simulink model "Airbag_donePrev"  (R2020b)
settings: Solver=VariableStepAuto  StartTime=0.0  StopTime=10  RelTol=1e-3
libraries: simulink x4
settings Model: Creator=HP  LastModifiedBy=HP

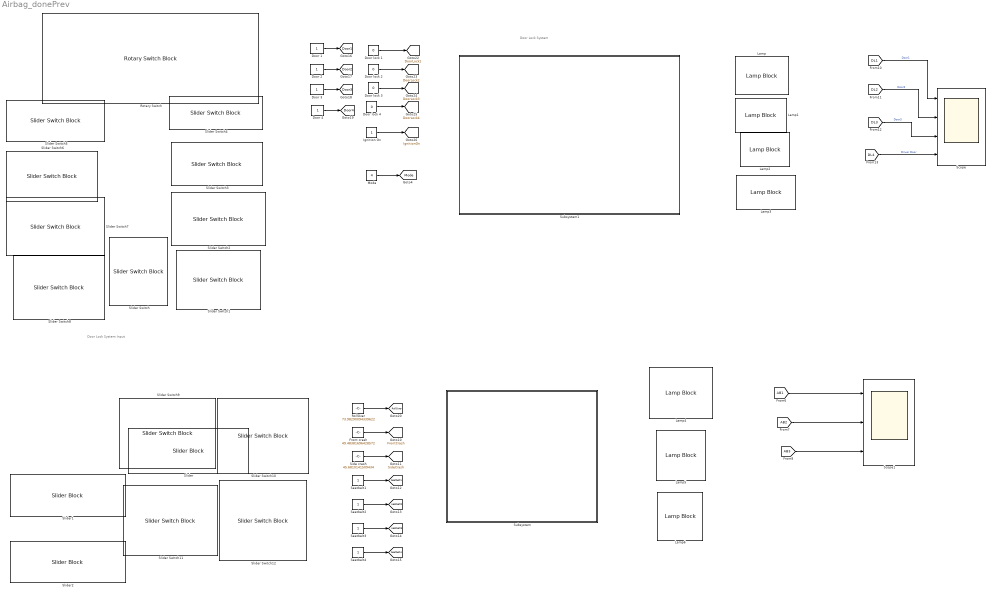
== system Airbag_donePrev ==
  note: Door Lock System
  note: Door Lock System Input
  Door {1..4} (4 alike) : Constant
  Door lock {1..4} (4 alike) : Constant  Value=0
  Front crash : Constant  Value=49.48381696428572
  Ignition On : Constant
  Lamp{,1..6} (7 alike) : LampBlock
  Mode : Constant  Value=4
  RollOver : Constant  Value=73.98290094339622
  Rotary Switch : RotarySwitchBlock
      settings: Values={{'Safety lock', 'Automatic Lock', 'Lock Out Protection', 'Driver Control Lock', 'Driver Control Unlock'}, [0 1 2 3 4]}
  Scope : Scope  NumInputPorts=4
  Scope1 : Scope  NumInputPorts=3
  Seatbelt{1..4} (4 alike) : Constant
  Side crash : Constant  Value=45.6810141509434
  Slider : SliderBlock
  Slider Switch{,1..12} (13 alike) : SliderSwitchBlock
      settings: Values={{'Off', 'On'}, [0 1]}
  Slider1 : SliderBlock
  Slider2 : SliderBlock
  Subsystem : Subsystem
  Subsystem1 : Subsystem
  tag scope: Door1=global, Door2=global, Door3=global, Door4=global, DoorLock1=global, DoorLock2=global, DoorLock3=global, DoorLock4=global, FrontCrash=global, IgnitionOn=global, Mode=global, RollOver=global, Seatbelt1=global, Seatbelt4=global, SideCrash=global, seatbelt2=global, seatbelt3=global
  wires:
  RollOver/1 -> [RollOver]
  Seatbelt3/1 -> [seatbelt3]
  Mode/1 -> [Mode]
  Seatbelt4/1 -> [Seatbelt4]
  Seatbelt2/1 -> [seatbelt2]
  [DL1] -> Scope/1  "Door1"
  Seatbelt1/1 -> [Seatbelt1]
  [DL4] -> Scope/4  "Driver Door"
  Side crash/1 -> [SideCrash]
  [DL2] -> Scope/2  "Door2"
  [AB1] -> Scope1/1
  [DL3] -> Scope/3  "Door3"
  [AB3] -> Scope1/3
  Front crash/1 -> [FrontCrash]
  [AB2] -> Scope1/2
  Door 3/1 -> [Door3]
  Ignition On/1 -> [IgnitionOn]
  Door lock 2/1 -> [DoorLock2]
  Door lock 3/1 -> [DoorLock3]
  Door lock 1/1 -> [DoorLock1]
  Door lock 4/1 -> [DoorLock4]
  Door 1/1 -> [Door1]
  Door 2/1 -> [Door2]
  Door 4/1 -> [Door4]

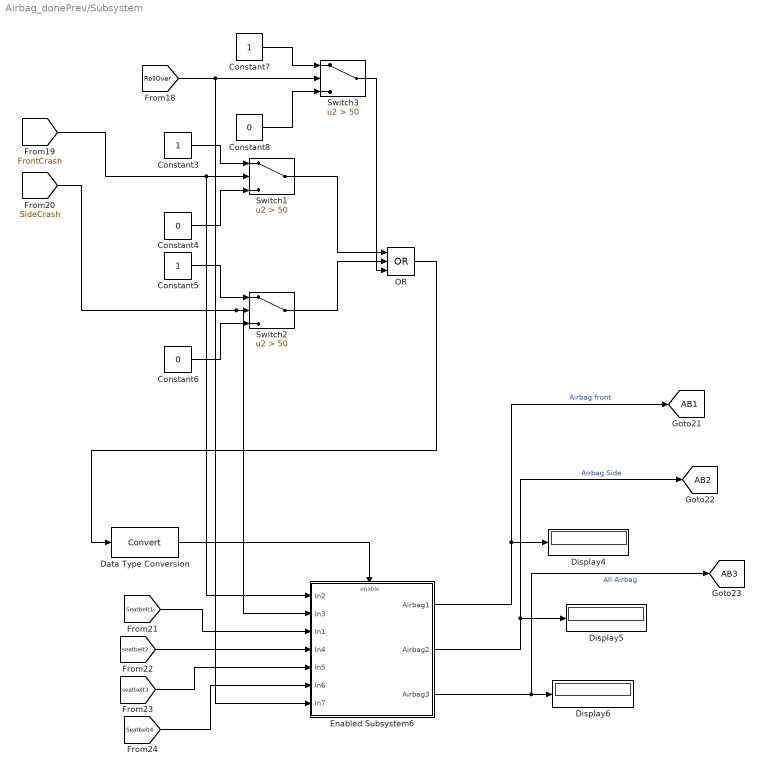
== system Airbag_donePrev/Subsystem ==
  Constant3 : Constant
  Constant4 : Constant  Value=0
  Constant5 : Constant
  Constant6 : Constant  Value=0
  Constant7 : Constant
  Constant8 : Constant  Value=0
  Data Type Conversion : DataTypeConversion
  Display4 : Display
  Display5 : Display
  Display6 : Display
  Enabled Subsystem6 : Subsystem  TreatAsAtomicUnit=on
  OR : Logic  Operator=OR  Inputs=3  IconShape=distinctive  AllPortsSameDT=off  OutDataTypeStr=boolean
  Switch1 : Switch  Criteria=u2 > Threshold  Threshold=50
  Switch2 : Switch  Criteria=u2 > Threshold  Threshold=50
  Switch3 : Switch  Criteria=u2 > Threshold  Threshold=50
  tag scope: AB1=global, AB2=global, AB3=global
  wires:
  Enabled Subsystem6/2(Airbag2) -> [AB2], Display5/1  "Airbag Side"
  Constant7/1 -> Switch3/1
  [Seatbelt4] -> Enabled Subsystem6/6(In6)
  Enabled Subsystem6/3(Airbag3) -> [AB3], Display6/1  "All Airbag"
  [RollOver] -> Enabled Subsystem6/7(In7), Switch3/2
  [seatbelt3] -> Enabled Subsystem6/5(In5)
  [SideCrash] -> Enabled Subsystem6/2(In3), Switch2/2
  Enabled Subsystem6/1(Airbag1) -> [AB1], Display4/1  "Airbag front"
  Data Type Conversion/1 -> Enabled Subsystem6/Enable
  [Seatbelt1] -> Enabled Subsystem6/3(In1)
  Switch3/1 -> OR/3
  Constant5/1 -> Switch2/1
  OR/1 -> Data Type Conversion/1
  Switch1/1 -> OR/1
  Constant6/1 -> Switch2/3
  [FrontCrash] -> Enabled Subsystem6/1(In2), Switch1/2
  Constant8/1 -> Switch3/3
  Switch2/1 -> OR/2
  [seatbelt2] -> Enabled Subsystem6/4(In4)
  Constant3/1 -> Switch1/1
  Constant4/1 -> Switch1/3

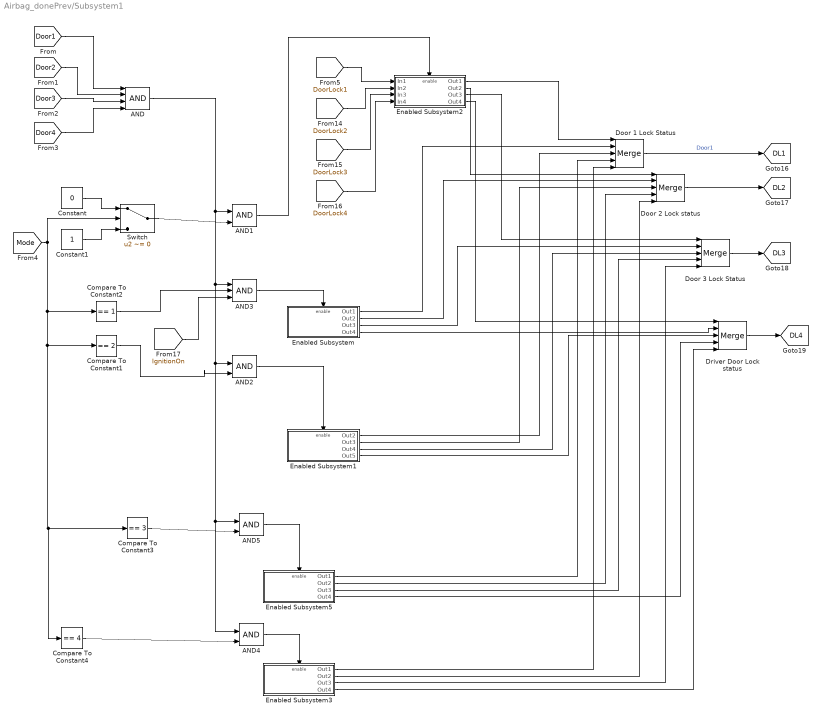
== system Airbag_donePrev/Subsystem1 ==
  AND : Logic  Inputs=4  IconShape=distinctive  AllPortsSameDT=off  OutDataTypeStr=boolean
  AND{1..2,4..5} (4 alike) : Logic  IconShape=distinctive  AllPortsSameDT=off  OutDataTypeStr=boolean
  AND3 : Logic  Inputs=3  IconShape=distinctive  AllPortsSameDT=off  OutDataTypeStr=boolean
  Compare To Constant1 : simulink/Logic and Bit Operations/Compare To Constant  relop===  const=2  OutDataTypeStr=boolean
  Compare To Constant2 : simulink/Logic and Bit Operations/Compare To Constant  relop===  const=1  OutDataTypeStr=boolean
  Compare To Constant3 : simulink/Logic and Bit Operations/Compare To Constant  relop===  const=3  OutDataTypeStr=boolean
  Compare To Constant4 : simulink/Logic and Bit Operations/Compare To Constant  relop===  const=4  OutDataTypeStr=boolean
  Constant : Constant  Value=0
  Constant1 : Constant
  Door 1 Lock Status : Merge  Inputs=5
  Door 2 Lock status : Merge  Inputs=5
  Door 3 Lock Status : Merge  Inputs=5
  "Driver Door Lock status " : Merge  Inputs=5
  Enabled Subsystem : Subsystem  TreatAsAtomicUnit=on
  Enabled Subsystem1 : Subsystem  TreatAsAtomicUnit=on
  Enabled Subsystem2 : Subsystem  TreatAsAtomicUnit=on
  Enabled Subsystem3 : Subsystem  TreatAsAtomicUnit=on
  Enabled Subsystem5 : Subsystem  TreatAsAtomicUnit=on
  Switch : Switch  Criteria=u2 ~= 0
  tag scope: DL1=global, DL2=global, DL3=global, DL4=global
  wires:
  [IgnitionOn] -> AND3/3
  "Driver Door Lock status "/1 -> [DL4]
  Enabled Subsystem5/1(Out1) -> Door 1 Lock Status/4
  AND1/1 -> Enabled Subsystem2/Enable
  Enabled Subsystem5/2(Out2) -> Door 2 Lock status/4
  Door 1 Lock Status/1 -> [DL1]  "Door1"
  [DoorLock2] -> Enabled Subsystem2/2(In2)
  Enabled Subsystem1/2(Out3) -> Door 2 Lock status/3
  Enabled Subsystem2/1(Out1) -> Door 1 Lock Status/1
  Enabled Subsystem2/2(Out2) -> Door 2 Lock status/1
  Enabled Subsystem1/1(Out2) -> Door 1 Lock Status/3
  AND5/1 -> Enabled Subsystem5/Enable
  [Door3] -> AND/3
  [Door4] -> AND/4
  Compare To Constant2/1 -> AND3/2
  Door 2 Lock status/1 -> [DL2]
  AND/1 -> AND5/1, AND4/1, AND2/1, AND3/1, AND1/1
  Enabled Subsystem1/3(Out4) -> Door 3 Lock Status/3
  [Door2] -> AND/2
  Switch/1 -> AND1/2
  [DoorLock3] -> Enabled Subsystem2/3(In3)
  [Mode] -> Switch/2, Compare To Constant2/1, Compare To Constant1/1, Compare To Constant4/1, Compare To Constant3/1
  Constant/1 -> Switch/1
  [DoorLock4] -> Enabled Subsystem2/4(In4)
  Enabled Subsystem5/3(Out3) -> Door 3 Lock Status/4
  Enabled Subsystem5/4(Out4) -> "Driver Door Lock status "/4
  [DoorLock1] -> Enabled Subsystem2/1(In1)
  Compare To Constant3/1 -> AND5/2
  Door 3 Lock Status/1 -> [DL3]
  Enabled Subsystem2/4(Out4) -> "Driver Door Lock status "/1
  Enabled Subsystem/2(Out2) -> Door 2 Lock status/2
  Enabled Subsystem/4(Out4) -> "Driver Door Lock status "/2
  Enabled Subsystem/1(Out1) -> Door 1 Lock Status/2
  [Door1] -> AND/1
  Constant1/1 -> Switch/3
  Enabled Subsystem2/3(Out3) -> Door 3 Lock Status/1
  Enabled Subsystem1/4(Out5) -> "Driver Door Lock status "/3
  Enabled Subsystem/3(Out3) -> Door 3 Lock Status/2
  Compare To Constant1/1 -> AND2/2
  AND3/1 -> Enabled Subsystem/Enable
  AND2/1 -> Enabled Subsystem1/Enable
  AND4/1 -> Enabled Subsystem3/Enable
  Compare To Constant4/1 -> AND4/2
  Enabled Subsystem3/4(Out4) -> "Driver Door Lock status "/5
  Enabled Subsystem3/3(Out3) -> Door 3 Lock Status/5
  Enabled Subsystem3/2(Out2) -> Door 2 Lock status/5
  Enabled Subsystem3/1(Out1) -> Door 1 Lock Status/5

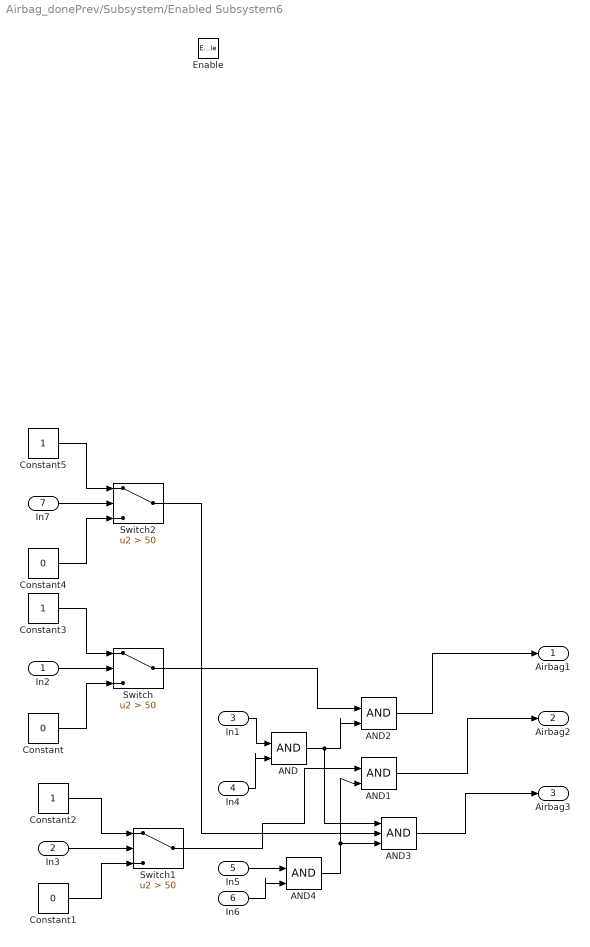
== system Airbag_donePrev/Subsystem/Enabled Subsystem6 ==
  In2 : Inport
  In3 : Inport  Port=2
  In1 : Inport  Port=3
  In4 : Inport  Port=4
  In5 : Inport  Port=5
  In6 : Inport  Port=6
  In7 : Inport  Port=7
  Enable : EnablePort
  AND{,1..2,4} (4 alike) : Logic  IconShape=distinctive  AllPortsSameDT=off  OutDataTypeStr=boolean
  AND3 : Logic  Inputs=3  IconShape=distinctive  AllPortsSameDT=off  OutDataTypeStr=boolean
  Constant : Constant  Value=0
  Constant1 : Constant  Value=0
  Constant2 : Constant
  Constant3 : Constant
  Constant4 : Constant  Value=0
  Constant5 : Constant
  Switch : Switch  Criteria=u2 > Threshold  Threshold=50
  Switch1 : Switch  Criteria=u2 > Threshold  Threshold=50
  Switch2 : Switch  Criteria=u2 > Threshold  Threshold=50
  Airbag1 : Outport
  Airbag2 : Outport  Port=2
  Airbag3 : Outport  Port=3
  wires:
  Constant2/1 -> Switch1/1
  In2/1 -> Switch/2
  Constant/1 -> Switch/3
  In3/1 -> Switch1/2
  Constant1/1 -> Switch1/3
  Constant3/1 -> Switch/1
  Switch/1 -> AND2/1
  AND2/1 -> Airbag1/1
  AND1/1 -> Airbag2/1
  AND3/1 -> Airbag3/1
  Switch1/1 -> AND1/1
  In1/1 -> AND/1
  In4/1 -> AND/2
  AND/1 -> AND3/1, AND2/2
  In5/1 -> AND4/1
  In6/1 -> AND4/2
  AND4/1 -> AND3/3, AND1/2
  In7/1 -> Switch2/2
  Constant4/1 -> Switch2/3
  Constant5/1 -> Switch2/1
  Switch2/1 -> AND3/2

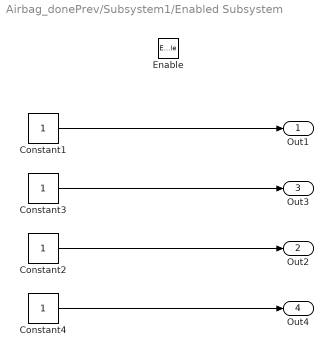
== system Airbag_donePrev/Subsystem1/Enabled Subsystem ==
  Enable : EnablePort
  Constant{1..4} (4 alike) : Constant
  Out1 : Outport
  Out2 : Outport  Port=2
  Out3 : Outport  Port=3
  Out4 : Outport  Port=4
  wires:
  Constant1/1 -> Out1/1
  Constant2/1 -> Out2/1
  Constant3/1 -> Out3/1
  Constant4/1 -> Out4/1

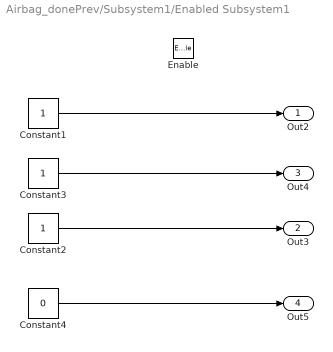
== system Airbag_donePrev/Subsystem1/Enabled Subsystem1 ==
  Enable : EnablePort
  Constant1 : Constant
  Constant2 : Constant
  Constant3 : Constant
  Constant4 : Constant  Value=0
  Out2 : Outport
  Out3 : Outport  Port=2
  Out4 : Outport  Port=3
  Out5 : Outport  Port=4
  wires:
  Constant2/1 -> Out3/1
  Constant3/1 -> Out4/1
  Constant1/1 -> Out2/1
  Constant4/1 -> Out5/1

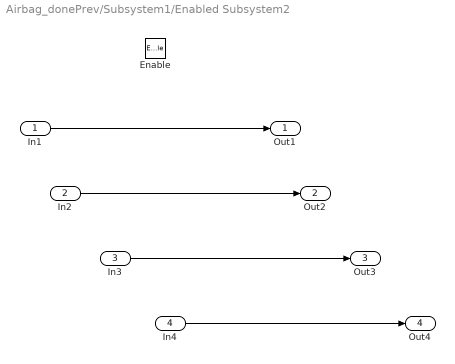
== system Airbag_donePrev/Subsystem1/Enabled Subsystem2 ==
  In1 : Inport
  In2 : Inport  Port=2
  In3 : Inport  Port=3
  In4 : Inport  Port=4
  Enable : EnablePort
  Out1 : Outport
  Out2 : Outport  Port=2
  Out3 : Outport  Port=3
  Out4 : Outport  Port=4
  wires:
  In1/1 -> Out1/1
  In2/1 -> Out2/1
  In3/1 -> Out3/1
  In4/1 -> Out4/1

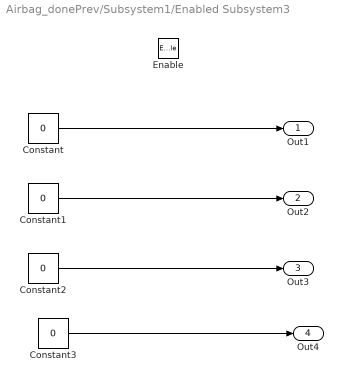
== system Airbag_donePrev/Subsystem1/Enabled Subsystem3 ==
  Enable : EnablePort
  Constant{,1..3} (4 alike) : Constant  Value=0
  Out1 : Outport
  Out2 : Outport  Port=2
  Out3 : Outport  Port=3
  Out4 : Outport  Port=4
  wires:
  Constant/1 -> Out1/1
  Constant1/1 -> Out2/1
  Constant2/1 -> Out3/1
  Constant3/1 -> Out4/1

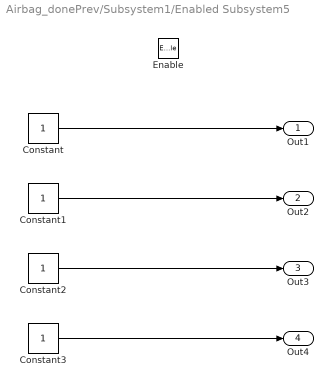
== system Airbag_donePrev/Subsystem1/Enabled Subsystem5 ==
  Enable : EnablePort
  Constant{,1..3} (4 alike) : Constant
  Out1 : Outport
  Out2 : Outport  Port=2
  Out3 : Outport  Port=3
  Out4 : Outport  Port=4
  wires:
  Constant/1 -> Out1/1
  Constant1/1 -> Out2/1
  Constant2/1 -> Out3/1
  Constant3/1 -> Out4/1
